simulink model "gm_HDL_pfc_gold_fi_og_vnl"  (R2024b)
settings: Solver=FixedStepDiscrete  StartTime=0.0  StopTime=.2  RelTol=1e-3
InitFcn:
  | fidelity_pfc_vals;
  | nbits=(2^12)-2;
  | load('C:\Users\Angel\Desktop\hil\pfc3ph\matlab\sim\sschdl\pfc_desktop\stateSpaceParameters.mat');
undefined symbols (not defined in the file or in its folder): a, b, c, DiscIntNeverNeededParam, fsw, Gs, s, stateSpaceParameters_1, t_ss, tsw
libraries: simulink x47, hdlmdlgenlib x24, hdlsllib x10, mcbcontrolslib x5, dspsrcs4 x3, slpidlib x2, hdlssclib x2, spsSVPWMGenerator2LevelLib x1, spsPLL3phLib x1, fillib x1
(part 2 of 5)

== system gm_HDL_pfc_gold_fi_og_vnl/Subsystem1/ctrl_pwm/PI_CTRL ==
  id : Inport
  iq : Inport  Port=2
  Add3 : Sum  Inputs=+-
  Add4 : Sum  Inputs=+-
  Constant : Constant  Value=0  SampleTime=t_ss
  Constant1 : Constant  Value=-4  SampleTime=t_ss
  Vd_ctrl : slpidlib/PID Controller  Controller=PI  Form=Parallel  TimeDomain=Discrete-time  UseExternalTs=off  SampleTime=-1  IntegratorMethod=Backward Euler  FilterMethod=Forward Euler  ControllerParametersSource=internal  P=-1.8  I=-.15  UseKiTs=off  D=0  UseExternalDerivativeSource=off  N=100  UseFilter=on  TunerSelectOption=Transfer Function Based (PID Tuner App)  InitialConditionSource=internal  InitialConditionForIntegrator=0  InitialConditionForFilter=0  DifferentiatorICPrevScaledInput=0  ExternalReset=none  TrackingMode=off  Kt=1  LimitOutput=off  SatLimitsSource=internal  UpperSaturationLimit=5e2  LowerSaturationLimit=-5e2  LinearizeAsGain=on  AntiWindupMode=clamping  Kb=1  LimitIntegrator=off  UpperIntegratorSaturationLimit=inf  LowerIntegratorSaturationLimit=-inf  POutMin=[]  POutMax=[]  IOutMin=[]  IOutMax=[]  DOutMin=[]  DOutMax=[]  NOutMin=[]  NOutMax=[]  SumOutMin=[]  SumOutMax=[]  SaturationOutMin=[]  SaturationOutMax=[]  PParamMin=[]  PParamMax=[]  IParamMin=[]  IParamMax=[]  DParamMin=[]  DParamMax=[]  NParamMin=[]  NParamMax=[]  KbParamMin=[]  KbParamMax=[]  KtParamMin=[]  KtParamMax=[]  KbOutMin=[]  KbOutMax=[]  KtOutMin=[]  KtOutMax=[]  IntegratorOutMin=[]  IntegratorOutMax=[]  FilterOutMin=[]  FilterOutMax=[]  SumI1OutMin=[]  SumI1OutMax=[]  SumI2OutMin=[]  SumI2OutMax=[]  SumI3OutMin=[]  SumI3OutMax=[]  SumI4OutMin=[]  SumI4OutMax=[]  SumDOutMin=[]  SumDOutMax=[]  DifferentiatorOutMin=[]  DifferentiatorOutMax=[]  FilterDiffOutCoefMin=[]  FilterDiffOutCoefMax=[]  ReciprocalOutMin=[]  ReciprocalOutMax=[]  SumDenOutMin=[]  SumDenOutMax=[]  SumNumOutMin=[]  SumNumOutMax=[]  DivideOutMin=[]  DivideOutMax=[]  UdiffTsProdOutMin=[]  UdiffTsProdOutMax=[]  NTsProdOutMin=[]  NTsProdOutMax=[]  UintegralTsProdOutMin=[]  UintegralTsProdOutMax=[]  UngainTsProdOutMin=[]  UngainTsProdOutMax=[]  ClampingZeroOutDataTypeStr=Inherit: Inherit via back propagation  ClampingZeroOutMin=[]  ClampingZeroOutMax=[]  FilterDenConstantOutDataTypeStr=Inherit: Inherit via back propagation  FilterDenConstantOutMin=[]  FilterDenConstantOutMax=[]  PCopyOutDataTypeStr=Inherit: Inherit via back propagation  PCopyOutMin=[]  PCopyOutMax=[]  NCopyOutDataTypeStr=Inherit: Inherit via back propagation  NCopyOutMin=[]  NCopyOutMax=[]  IntegratorContinuousStateAttributes=''  IntegratorStateMustResolveToSignalObject=off  IntegratorRTWStateStorageClass=Auto  FilterContinuousStateAttributes=''  FilterStateMustResolveToSignalObject=off  FilterRTWStateStorageClass=Auto  ParallelPVariant=InternalParameters  IdealPVariant=Disabled  IVariant=InternalParameters  DVariant=Disabled  IntegratorVariant=Discrete  SatVariant=Disabled  AWVariant=Passthrough  PCopyVariant=Disabled  TRVariant=Disabled  FdbkBlocksVariant=Forward  IdealPFdbkVariant=Disabled  SatFdbkVariant=Disabled  DerivativeFilterVariant=Disabled  NVariant=Disabled  NCopyVariant=Disabled_SignalSpec  FilterICVariant=Disabled  IntegratorICVariant=InternalICs  ExternalResetVariant=Disabled  TRSumVariant=Passthrough  SumFdbkVariant=Disabled  SumVariant=Sum_PI  TsampFilterVariant=InternalTs  TsampNgainVariant=Passthrough  TsampIntegralVariant=Disabled_SignalSpec  ExternalSaturationOutDataTypeStr=Inherit: Same as second input  DerivativeSourceVariant=Disabled  PreIntVariant=InternalPreInt
  Vq_ctrl : slpidlib/PID Controller  Controller=PI  Form=Parallel  TimeDomain=Discrete-time  UseExternalTs=off  SampleTime=-1  IntegratorMethod=Backward Euler  FilterMethod=Forward Euler  ControllerParametersSource=internal  P=-2  I=-.2  UseKiTs=off  D=0  UseExternalDerivativeSource=off  N=100  UseFilter=on  TunerSelectOption=Transfer Function Based (PID Tuner App)  InitialConditionSource=internal  InitialConditionForIntegrator=0  InitialConditionForFilter=0  DifferentiatorICPrevScaledInput=0  ExternalReset=none  TrackingMode=off  Kt=1  LimitOutput=off  SatLimitsSource=internal  UpperSaturationLimit=5e2  LowerSaturationLimit=-5e2  LinearizeAsGain=on  AntiWindupMode=clamping  Kb=1  LimitIntegrator=off  UpperIntegratorSaturationLimit=inf  LowerIntegratorSaturationLimit=-inf  POutMin=[]  POutMax=[]  IOutMin=[]  IOutMax=[]  DOutMin=[]  DOutMax=[]  NOutMin=[]  NOutMax=[]  SumOutMin=[]  SumOutMax=[]  SaturationOutMin=[]  SaturationOutMax=[]  PParamMin=[]  PParamMax=[]  IParamMin=[]  IParamMax=[]  DParamMin=[]  DParamMax=[]  NParamMin=[]  NParamMax=[]  KbParamMin=[]  KbParamMax=[]  KtParamMin=[]  KtParamMax=[]  KbOutMin=[]  KbOutMax=[]  KtOutMin=[]  KtOutMax=[]  IntegratorOutMin=[]  IntegratorOutMax=[]  FilterOutMin=[]  FilterOutMax=[]  SumI1OutMin=[]  SumI1OutMax=[]  SumI2OutMin=[]  SumI2OutMax=[]  SumI3OutMin=[]  SumI3OutMax=[]  SumI4OutMin=[]  SumI4OutMax=[]  SumDOutMin=[]  SumDOutMax=[]  DifferentiatorOutMin=[]  DifferentiatorOutMax=[]  FilterDiffOutCoefMin=[]  FilterDiffOutCoefMax=[]  ReciprocalOutMin=[]  ReciprocalOutMax=[]  SumDenOutMin=[]  SumDenOutMax=[]  SumNumOutMin=[]  SumNumOutMax=[]  DivideOutMin=[]  DivideOutMax=[]  UdiffTsProdOutMin=[]  UdiffTsProdOutMax=[]  NTsProdOutMin=[]  NTsProdOutMax=[]  UintegralTsProdOutMin=[]  UintegralTsProdOutMax=[]  UngainTsProdOutMin=[]  UngainTsProdOutMax=[]  ClampingZeroOutDataTypeStr=Inherit: Inherit via back propagation  ClampingZeroOutMin=[]  ClampingZeroOutMax=[]  FilterDenConstantOutDataTypeStr=Inherit: Inherit via back propagation  FilterDenConstantOutMin=[]  FilterDenConstantOutMax=[]  PCopyOutDataTypeStr=Inherit: Inherit via back propagation  PCopyOutMin=[]  PCopyOutMax=[]  NCopyOutDataTypeStr=Inherit: Inherit via back propagation  NCopyOutMin=[]  NCopyOutMax=[]  IntegratorContinuousStateAttributes=''  IntegratorStateMustResolveToSignalObject=off  IntegratorRTWStateStorageClass=Auto  FilterContinuousStateAttributes=''  FilterStateMustResolveToSignalObject=off  FilterRTWStateStorageClass=Auto  ParallelPVariant=InternalParameters  IdealPVariant=Disabled  IVariant=InternalParameters  DVariant=Disabled  IntegratorVariant=Discrete  SatVariant=Disabled  AWVariant=Passthrough  PCopyVariant=Disabled  TRVariant=Disabled  FdbkBlocksVariant=Forward  IdealPFdbkVariant=Disabled  SatFdbkVariant=Disabled  DerivativeFilterVariant=Disabled  NVariant=Disabled  NCopyVariant=Disabled_SignalSpec  FilterICVariant=Disabled  IntegratorICVariant=InternalICs  ExternalResetVariant=Disabled  TRSumVariant=Passthrough  SumFdbkVariant=Disabled  SumVariant=Sum_PI  TsampFilterVariant=InternalTs  TsampNgainVariant=Passthrough  TsampIntegralVariant=Disabled_SignalSpec  ExternalSaturationOutDataTypeStr=Inherit: Same as second input  DerivativeSourceVariant=Disabled  PreIntVariant=InternalPreInt
  Vd_inductor : Outport
  Vq_inductor : Outport  Port=2
  wires:
  Add3/1 -> Vd_ctrl/1  "error_id"
  id/1 -> Add3/2
  Constant/1 -> Add3/1
  iq/1 -> Add4/2
  Add4/1 -> Vq_ctrl/1  "error_iq"
  Vd_ctrl/1 -> Vd_inductor/1
  Vq_ctrl/1 -> Vq_inductor/1
  Constant1/1 -> Add4/1

== system gm_HDL_pfc_gold_fi_og_vnl/Subsystem1/ctrl_pwm/SVPWM ==
  Vd_inductor : Inport
  angle : Inport  Port=2
  Vq_inductor : Inport  Port=3
  Cos : Trigonometry  Operator=cos
  Inverse Park Transform : mcbcontrolslib/Inverse Park Transform  PhaseInput=Two inputs  AxisAlignment=D-axis  ThetaInput=Sine and Cosine electrical position  AngleInput=Per-unit  N_points=1024
  SVPWM Generator (2-Level) : spsSVPWMGenerator2LevelLib/SVPWM Generator (2-Level)  InputType=alpha-beta components  SwitchingPattern=Pattern #1  Fc=fsw*1e3  ParUref=[0.8 -30 50]  Ts=t_ss
  Sin : Trigonometry
  P : Outport
  wires:
  Vd_inductor/1 -> Inverse Park Transform/1
  Vq_inductor/1 -> Inverse Park Transform/2
  Inverse Park Transform/2 -> SVPWM Generator (2-Level)/2  "Vbet_indc"
  Sin/1 -> Inverse Park Transform/3
  Cos/1 -> Inverse Park Transform/4
  Inverse Park Transform/1 -> SVPWM Generator (2-Level)/1  "Valp_indc"
  angle/1 -> Cos/1, Sin/1
  SVPWM Generator (2-Level)/1 -> P/1

== system gm_HDL_pfc_gold_fi_og_vnl/Subsystem1/ctrl_pwm/transforms ==
  a : Inport
  b : Inport  Port=2
  In3 : Inport  Port=3
  In4 : Inport  Port=4
  In5 : Inport  Port=5
  Claro-Parl Transform : Subsystem  Commented=on
  Claro-Parl Transform1 : Subsystem
  Delay : Delay  DelayLength=1
  Delay1 : Delay  DelayLength=1
  Mux : Mux  Inputs=3
  PLL (3ph) : spsPLL3phLib/PLL (3ph)  Fmin=50  Par_Init=[0, 50]  ParK=[180,3200,1]  TcD=1e-4  MaxRateChangeFreq=12  FilterCutOffFreq=25  Ts=t_ss  AGC=on
  Terminator : Terminator
  id : Outport
  iq : Outport  Port=2
  angle : Outport  Port=3
  wires:
  Mux/1 -> PLL (3ph)/1
  PLL (3ph)/2 -> angle/1, Claro-Parl Transform1/3(wt), Claro-Parl Transform/3(wt)  "angle"
  PLL (3ph)/1 -> Terminator/1
  In3/1 -> Mux/1, Claro-Parl Transform/1(a)
  In5/1 -> Mux/3
  b/1 -> Delay1/1
  In4/1 -> Claro-Parl Transform/2(b), Mux/2
  a/1 -> Delay/1
  Delay/1 -> Claro-Parl Transform1/1(a)
  Delay1/1 -> Claro-Parl Transform1/2(b)
  Claro-Parl Transform/1(d) -> ?  "vd"
  Claro-Parl Transform/2(q) -> ?  "vq"
  Claro-Parl Transform1/1(d) -> id/1  "id"
  Claro-Parl Transform1/2(q) -> iq/1  "iq"

== system gm_HDL_pfc_gold_fi_og_vnl/simscape_system/simscape_system/FET_CTRL ==
  vs : Inport  OutDataTypeStr=fixdt(1, 18, 6)  PortDimensions=[6]  SampleTime=1.38600138600139e-08
  is : Inport  Port=2  OutDataTypeStr=fixdt(1, 18, 6)  PortDimensions=[6]  SampleTime=1.38600138600139e-08
  G : Inport  Port=3  OutDataTypeStr=boolean  PortDimensions=[6]  SampleTime=1.38600138600139e-08
  sch_ctr_36 : Inport  Port=4  OutDataTypeStr=fixdt(0, 6, 0)  SampleTime=1.38600138600139e-08
  Discrete-Time Integrator_reg : RateTransition  InitialCondition=double(0)  OutPortSampleTimeOpt=Multiple of input port sample time  OutPortSampleTimeMultiple=37
  Discrete-Time Integrator_reg_absorbed : Delay  DelayLength=0
  crp_temp_streamed : Subsystem
  in0_repeat : RateTransition  Integrity=off  Deterministic=off  OutPortSampleTimeOpt=Multiple of input port sample time  OutPortSampleTimeMultiple=1/37
  ic : Outport  SampleTime=1.38600138600139e-08
  wires:
  Discrete-Time Integrator_reg_absorbed/1 -> in0_repeat/1
  crp_temp_streamed/2(out1) -> ic/1
  sch_ctr_36/1 -> crp_temp_streamed/5(enb_counter)
  Discrete-Time Integrator_reg/1 -> Discrete-Time Integrator_reg_absorbed/1
  is/1 -> crp_temp_streamed/4(in3)
  vs/1 -> crp_temp_streamed/3(in2)
  crp_temp_streamed/1(out0) -> Discrete-Time Integrator_reg/1
  in0_repeat/1 -> crp_temp_streamed/1(in0)
  G/1 -> crp_temp_streamed/2(in1)

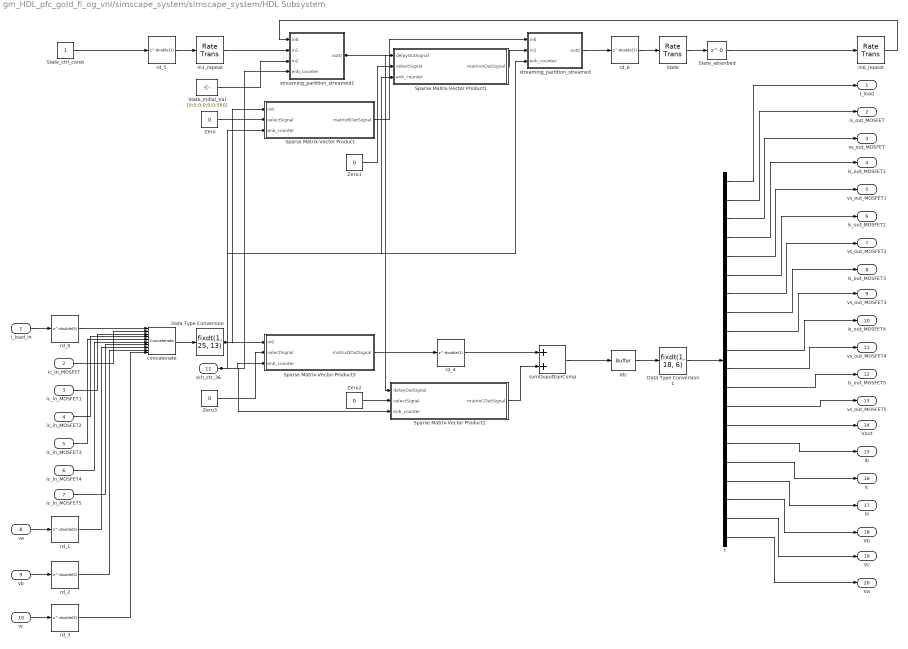
== system gm_HDL_pfc_gold_fi_og_vnl/simscape_system/simscape_system/HDL Subsystem ==
  I_load_in : Inport  OutDataTypeStr=fixdt(1, 18, 8)  PortDimensions=1  SampleTime=1.38600138600139e-08
  ic_in_MOSFET : Inport  Port=2  OutDataTypeStr=fixdt(1, 18, 8)  PortDimensions=1  SampleTime=1.38600138600139e-08
  ic_in_MOSFET1 : Inport  Port=3  OutDataTypeStr=fixdt(1, 18, 8)  PortDimensions=1  SampleTime=1.38600138600139e-08
  ic_in_MOSFET2 : Inport  Port=4  OutDataTypeStr=fixdt(1, 18, 8)  PortDimensions=1  SampleTime=1.38600138600139e-08
  ic_in_MOSFET3 : Inport  Port=5  OutDataTypeStr=fixdt(1, 18, 8)  PortDimensions=1  SampleTime=1.38600138600139e-08
  ic_in_MOSFET4 : Inport  Port=6  OutDataTypeStr=fixdt(1, 18, 8)  PortDimensions=1  SampleTime=1.38600138600139e-08
  ic_in_MOSFET5 : Inport  Port=7  OutDataTypeStr=fixdt(1, 18, 8)  PortDimensions=1  SampleTime=1.38600138600139e-08
  va : Inport  Port=8  OutDataTypeStr=fixdt(1, 18, 8)  PortDimensions=1  SampleTime=1.38600138600139e-08
  vb : Inport  Port=9  OutDataTypeStr=fixdt(1, 18, 8)  PortDimensions=1  SampleTime=1.38600138600139e-08
  vc : Inport  Port=10  OutDataTypeStr=fixdt(1, 18, 8)  PortDimensions=1  SampleTime=1.38600138600139e-08
  sch_ctr_36 : Inport  Port=11  OutDataTypeStr=fixdt(0, 6, 0)  SampleTime=1.38600138600139e-08
  Data Type Conversion : DataTypeConversion  OutDataTypeStr=fixdt(1, 25, 13)  SampleTime=1.38600138600139e-08  SaturateOnIntegerOverflow=off  RndMeth=Floor
  Data Type Conversion1 : DataTypeConversion  OutDataTypeStr=fixdt(1, 18, 6)  SampleTime=1.38600138600139e-08  SaturateOnIntegerOverflow=off  RndMeth=Floor
  Sparse Matrix-Vector Product : Subsystem
  Sparse Matrix-Vector Product1 : Subsystem
  Sparse Matrix-Vector Product2 : Subsystem
  Sparse Matrix-Vector Product3 : Subsystem
  State : RateTransition  InitialCondition=double(0)  OutPortSampleTimeOpt=Multiple of input port sample time  OutPortSampleTimeMultiple=37
  State_Initial_Val : Constant  Value=[0;0;0;0;0;0;580]  OutDataTypeStr=fixdt(1, 25, 13)  SampleTime=1.38600138600139e-08
  State_absorbed : Delay  DelayLength=0
  State_ctrl_const : Constant  OutDataTypeStr=boolean  SampleTime=5.12820512820513e-07
  Zero{,1..3} (4 alike) : Constant  Value=0  OutDataTypeStr=boolean  SampleTime=1.38600138600139e-08
  concatenate : Concatenate  NumInputs=10
  dtc : hdlmdlgenlib/Buffer
  in0_repeat : RateTransition  Integrity=off  Deterministic=off  OutPortSampleTimeOpt=Multiple of input port sample time  OutPortSampleTimeMultiple=1/37
  in1_repeat : RateTransition  Integrity=off  Deterministic=off  OutPortSampleTimeOpt=Multiple of input port sample time  OutPortSampleTimeMultiple=1/37
  rd_{0..3} (4 alike) : Delay  DelayLength=double(5)  InitialCondition=0  SampleTime=1.38600138600139e-08
  rd_4 : Delay  DelayLength=double(1)  InitialCondition=0  SampleTime=1.38600138600139e-08
  rd_5 : Delay  DelayLength=double(1)  InitialCondition=0  SampleTime=5.12820512820513e-07
  rd_6 : Delay  DelayLength=double(1)  InitialCondition=0  SampleTime=1.38600138600139e-08
  streaming_partition_streamed : Subsystem
  streaming_partition_streamed1 : Subsystem
  sumOuputEqnComp : Sum  OutDataTypeStr=fixdt(1, 25, 13)  SampleTime=1.38600138600139e-08
  t : Demux  Outputs=20
  I_load : Outport  SampleTime=1.38600138600139e-08
  is_out_MOSFET : Outport  Port=2  SampleTime=1.38600138600139e-08
  vs_out_MOSFET : Outport  Port=3  SampleTime=1.38600138600139e-08
  is_out_MOSFET1 : Outport  Port=4  SampleTime=1.38600138600139e-08
  vs_out_MOSFET1 : Outport  Port=5  SampleTime=1.38600138600139e-08
  is_out_MOSFET2 : Outport  Port=6  SampleTime=1.38600138600139e-08
  vs_out_MOSFET2 : Outport  Port=7  SampleTime=1.38600138600139e-08
  is_out_MOSFET3 : Outport  Port=8  SampleTime=1.38600138600139e-08
  vs_out_MOSFET3 : Outport  Port=9  SampleTime=1.38600138600139e-08
  is_out_MOSFET4 : Outport  Port=10  SampleTime=1.38600138600139e-08
  vs_out_MOSFET4 : Outport  Port=11  SampleTime=1.38600138600139e-08
  is_out_MOSFET5 : Outport  Port=12  SampleTime=1.38600138600139e-08
  vs_out_MOSFET5 : Outport  Port=13  SampleTime=1.38600138600139e-08
  Vout : Outport  Port=14  SampleTime=1.38600138600139e-08
  Ib : Outport  Port=15  SampleTime=1.38600138600139e-08
  Ic : Outport  Port=16  SampleTime=1.38600138600139e-08
  Ia : Outport  Port=17  SampleTime=1.38600138600139e-08
  Vb : Outport  Port=18  SampleTime=1.38600138600139e-08
  Vc : Outport  Port=19  SampleTime=1.38600138600139e-08
  Va : Outport  Port=20  SampleTime=1.38600138600139e-08
  wires:
  in0_repeat/1 -> streaming_partition_streamed1/1(in0)
  t/14 -> Vout/1
  t/6 -> is_out_MOSFET2/1
  t/3 -> vs_out_MOSFET/1
  t/1 -> I_load/1
  State_absorbed/1 -> in0_repeat/1
  Data Type Conversion1/1 -> t/1
  State/1 -> State_absorbed/1
  dtc/1 -> Data Type Conversion1/1
  sumOuputEqnComp/1 -> dtc/1
  t/15 -> Ib/1
  rd_4/1 -> sumOuputEqnComp/1
  Sparse Matrix-Vector Product2/1(matrixCOutSignal) -> sumOuputEqnComp/2
  Sparse Matrix-Vector Product1/1(matrixAOutSignal) -> streaming_partition_streamed/2(in1)
  Zero2/1 -> Sparse Matrix-Vector Product2/2(selectSignal)
  Sparse Matrix-Vector Product/1(matrixBOutSignal) -> streaming_partition_streamed/1(in0)
  streaming_partition_streamed1/1(out0) -> Sparse Matrix-Vector Product2/1(delayOutSignal), Sparse Matrix-Vector Product1/1(delayOutSignal)
  Zero3/1 -> Sparse Matrix-Vector Product3/2(selectSignal)
  Data Type Conversion/1 -> Sparse Matrix-Vector Product/1(in0), Sparse Matrix-Vector Product3/1(in0)
  t/12 -> is_out_MOSFET5/1
  t/16 -> Ic/1
  Zero/1 -> Sparse Matrix-Vector Product/2(selectSignal)
  in1_repeat/1 -> streaming_partition_streamed1/2(in1)
  t/8 -> is_out_MOSFET3/1
  concatenate/1 -> Data Type Conversion/1
  t/2 -> is_out_MOSFET/1
  t/20 -> Va/1
  rd_5/1 -> in1_repeat/1
  rd_3/1 -> concatenate/10
  rd_2/1 -> concatenate/9
  t/18 -> Vb/1
  rd_1/1 -> concatenate/8
  t/19 -> Vc/1
  ic_in_MOSFET5/1 -> concatenate/7
  Zero1/1 -> Sparse Matrix-Vector Product1/2(selectSignal)
  ic_in_MOSFET4/1 -> concatenate/6
  streaming_partition_streamed/1(out0) -> rd_6/1
  ic_in_MOSFET3/1 -> concatenate/5
  ic_in_MOSFET2/1 -> concatenate/4
  Sparse Matrix-Vector Product3/1(matrixDOutSignal) -> rd_4/1
  ic_in_MOSFET1/1 -> concatenate/3
  sch_ctr_36/1 -> streaming_partition_streamed/3(enb_counter), Sparse Matrix-Vector Product/3(enb_counter), Sparse Matrix-Vector Product2/3(enb_counter), streaming_partition_streamed1/4(enb_counter), Sparse Matrix-Vector Product3/3(enb_counter), Sparse Matrix-Vector Product1/3(enb_counter)
  rd_6/1 -> State/1
  t/13 -> vs_out_MOSFET5/1
  t/17 -> Ia/1
  rd_0/1 -> concatenate/1
  ic_in_MOSFET/1 -> concatenate/2
  t/4 -> is_out_MOSFET1/1
  t/10 -> is_out_MOSFET4/1
  vc/1 -> rd_3/1
  State_Initial_Val/1 -> streaming_partition_streamed1/3(in2)
  va/1 -> rd_1/1
  t/9 -> vs_out_MOSFET3/1
  I_load_in/1 -> rd_0/1
  t/5 -> vs_out_MOSFET1/1
  t/7 -> vs_out_MOSFET2/1
  t/11 -> vs_out_MOSFET4/1
  vb/1 -> rd_2/1
  State_ctrl_const/1 -> rd_5/1

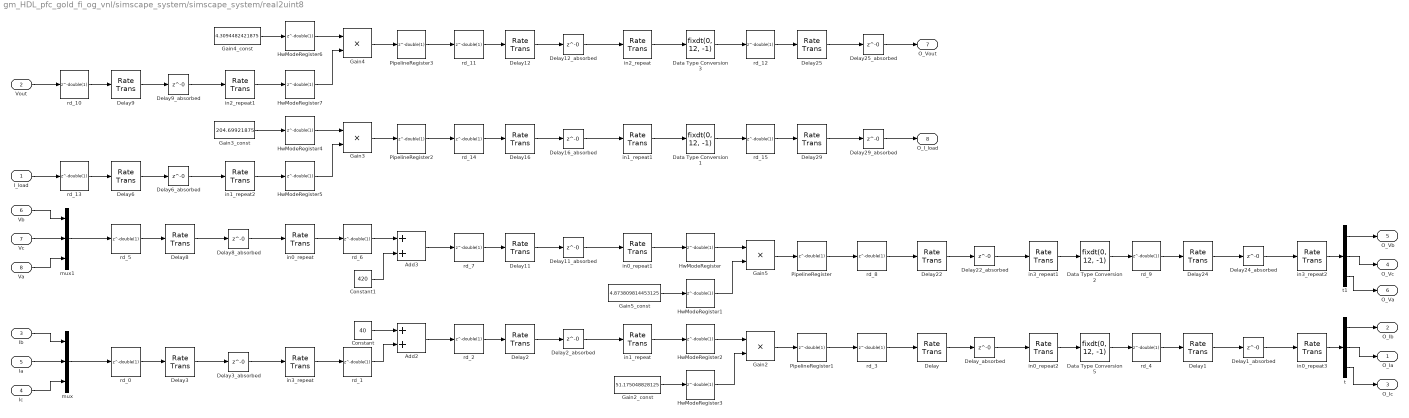
== system gm_HDL_pfc_gold_fi_og_vnl/simscape_system/simscape_system/real2uint8 ==
  I_load : Inport  OutDataTypeStr=fixdt(1, 18, 6)  PortDimensions=1  SampleTime=1.38600138600139e-08
  Vout : Inport  Port=2  OutDataTypeStr=fixdt(1, 18, 6)  PortDimensions=1  SampleTime=1.38600138600139e-08
  Ib : Inport  Port=3  OutDataTypeStr=fixdt(1, 18, 6)  PortDimensions=1  SampleTime=1.38600138600139e-08
  Ic : Inport  Port=4  OutDataTypeStr=fixdt(1, 18, 6)  PortDimensions=1  SampleTime=1.38600138600139e-08
  Ia : Inport  Port=5  OutDataTypeStr=fixdt(1, 18, 6)  PortDimensions=1  SampleTime=1.38600138600139e-08
  Vb : Inport  Port=6  OutDataTypeStr=fixdt(1, 18, 6)  PortDimensions=1  SampleTime=1.38600138600139e-08
  Vc : Inport  Port=7  OutDataTypeStr=fixdt(1, 18, 6)  PortDimensions=1  SampleTime=1.38600138600139e-08
  Va : Inport  Port=8  OutDataTypeStr=fixdt(1, 18, 6)  PortDimensions=1  SampleTime=1.38600138600139e-08
  Add2 : Sum  OutDataTypeStr=fixdt(1, 19, 6)  AccumDataTypeStr=fixdt(1, 19, 6)  SampleTime=1.38600138600139e-08
  Add3 : Sum  OutDataTypeStr=fixdt(1, 19, 6)  AccumDataTypeStr=fixdt(1, 19, 6)  SampleTime=1.38600138600139e-08
  Constant : Constant  Value=40  OutDataTypeStr=fixdt(1, 18, 6)  SampleTime=1.38600138600139e-08
  Constant1 : Constant  Value=420  OutDataTypeStr=fixdt(1, 18, 6)  SampleTime=1.38600138600139e-08
  Data Type Conversion{1..3,5} (4 alike) : DataTypeConversion  OutDataTypeStr=fixdt(0, 12, -1)  SampleTime=1.38600138600139e-08  SaturateOnIntegerOverflow=off  RndMeth=Floor
  Delay{,1..3,6,8..9,11..12,16,22,24..25,29} (14 alike) : RateTransition  InitialCondition=double(0)  OutPortSampleTimeOpt=Multiple of input port sample time  OutPortSampleTimeMultiple=37
  Delay11_absorbed : Delay  DelayLength=0
  Delay12_absorbed : Delay  DelayLength=0
  Delay16_absorbed : Delay  DelayLength=0
  Delay1_absorbed : Delay  DelayLength=0
  Delay22_absorbed : Delay  DelayLength=0
  Delay24_absorbed : Delay  DelayLength=0
  Delay25_absorbed : Delay  DelayLength=0
  Delay29_absorbed : Delay  DelayLength=0
  Delay2_absorbed : Delay  DelayLength=0
  Delay3_absorbed : Delay  DelayLength=0
  Delay6_absorbed : Delay  DelayLength=0
  Delay8_absorbed : Delay  DelayLength=0
  Delay9_absorbed : Delay  DelayLength=0
  Delay_absorbed : Delay  DelayLength=0
  Gain2 : Product  Inputs=**  OutDataTypeStr=fixdt(1, 38, 18)  SampleTime=1.38600138600139e-08
  Gain2_const : Constant  Value=51.175048828125  OutDataTypeStr=fixdt(1, 19, 12)  SampleTime=1.38600138600139e-08
  Gain3 : Product  Inputs=**  OutDataTypeStr=fixdt(1, 36, 15)  SampleTime=1.38600138600139e-08
  Gain3_const : Constant  Value=204.69921875  OutDataTypeStr=fixdt(1, 18, 9)  SampleTime=1.38600138600139e-08
  Gain4 : Product  Inputs=**  OutDataTypeStr=fixdt(1, 36, 20)  SampleTime=1.38600138600139e-08
  Gain4_const : Constant  Value=4.3094482421875  OutDataTypeStr=fixdt(1, 18, 14)  SampleTime=1.38600138600139e-08
  Gain5 : Product  Inputs=**  OutDataTypeStr=fixdt(1, 38, 21)  SampleTime=1.38600138600139e-08
  Gain5_const : Constant  Value=4.873809814453125  OutDataTypeStr=fixdt(1, 19, 15)  SampleTime=1.38600138600139e-08
  HwModeRegister{,1..7} (8 alike) : Delay  DelayLength=double(1)  InitialCondition=0  SampleTime=1.38600138600139e-08
  PipelineRegister{,1..3} (4 alike) : Delay  DelayLength=double(1)  InitialCondition=0  SampleTime=1.38600138600139e-08
  in0_repeat{,1..3} (4 alike) : RateTransition  Integrity=off  Deterministic=off  OutPortSampleTimeOpt=Multiple of input port sample time  OutPortSampleTimeMultiple=1/37
  in1_repeat : RateTransition  Integrity=off  Deterministic=off  OutPortSampleTimeOpt=Multiple of input port sample time  OutPortSampleTimeMultiple=1/37
  in1_repeat1 : RateTransition  Integrity=off  Deterministic=off  OutPortSampleTimeOpt=Multiple of input port sample time  OutPortSampleTimeMultiple=1/37
  in1_repeat2 : RateTransition  Integrity=off  Deterministic=off  OutPortSampleTimeOpt=Multiple of input port sample time  OutPortSampleTimeMultiple=1/37
  in2_repeat : RateTransition  Integrity=off  Deterministic=off  OutPortSampleTimeOpt=Multiple of input port sample time  OutPortSampleTimeMultiple=1/37
  in2_repeat1 : RateTransition  Integrity=off  Deterministic=off  OutPortSampleTimeOpt=Multiple of input port sample time  OutPortSampleTimeMultiple=1/37
  in3_repeat : RateTransition  Integrity=off  Deterministic=off  OutPortSampleTimeOpt=Multiple of input port sample time  OutPortSampleTimeMultiple=1/37
  in3_repeat1 : RateTransition  Integrity=off  Deterministic=off  OutPortSampleTimeOpt=Multiple of input port sample time  OutPortSampleTimeMultiple=1/37
  in3_repeat2 : RateTransition  Integrity=off  Deterministic=off  OutPortSampleTimeOpt=Multiple of input port sample time  OutPortSampleTimeMultiple=1/37
  mux : Mux  Inputs=3
  mux1 : Mux  Inputs=3
  rd_{0..15} (16 alike) : Delay  DelayLength=double(1)  InitialCondition=0  SampleTime=1.38600138600139e-08
  t : Demux  Outputs=3
  t1 : Demux  Outputs=3
  O_Ia : Outport  SampleTime=1.38600138600139e-08
  O_Ib : Outport  Port=2  SampleTime=1.38600138600139e-08
  O_Ic : Outport  Port=3  SampleTime=1.38600138600139e-08
  O_Vc : Outport  Port=4  SampleTime=1.38600138600139e-08
  O_Vb : Outport  Port=5  SampleTime=1.38600138600139e-08
  O_Va : Outport  Port=6  SampleTime=1.38600138600139e-08
  O_Vout : Outport  Port=7  SampleTime=5.12820512820513e-07
  O_I_load : Outport  Port=8  SampleTime=5.12820512820513e-07
  wires:
  t/3 -> O_Ic/1
  t/2 -> O_Ia/1
  t/1 -> O_Ib/1
  t1/3 -> O_Va/1
  t1/2 -> O_Vc/1
  t1/1 -> O_Vb/1
  in0_repeat3/1 -> t/1
  Delay1_absorbed/1 -> in0_repeat3/1
  Delay24_absorbed/1 -> in3_repeat2/1
  rd_4/1 -> Delay1/1
  rd_9/1 -> Delay24/1
  Data Type Conversion5/1 -> rd_4/1
  Data Type Conversion2/1 -> rd_9/1
  in0_repeat2/1 -> Data Type Conversion5/1
  in3_repeat1/1 -> Data Type Conversion2/1
  Delay_absorbed/1 -> in0_repeat2/1
  Delay22_absorbed/1 -> in3_repeat1/1
  Delay/1 -> Delay_absorbed/1
  Delay22/1 -> Delay22_absorbed/1
  rd_3/1 -> Delay/1
  rd_8/1 -> Delay22/1
  Delay29_absorbed/1 -> O_I_load/1
  Delay25_absorbed/1 -> O_Vout/1
  PipelineRegister1/1 -> rd_3/1
  Delay29/1 -> Delay29_absorbed/1
  Delay25/1 -> Delay25_absorbed/1
  Gain2/1 -> PipelineRegister1/1
  Gain5/1 -> PipelineRegister/1
  rd_15/1 -> Delay29/1
  rd_12/1 -> Delay25/1
  HwModeRegister2/1 -> Gain2/1
  HwModeRegister/1 -> Gain5/1
  Data Type Conversion3/1 -> rd_12/1
  Gain2_const/1 -> HwModeRegister3/1
  in2_repeat/1 -> Data Type Conversion3/1
  Gain5_const/1 -> HwModeRegister1/1
  Delay11_absorbed/1 -> in0_repeat1/1
  Data Type Conversion1/1 -> rd_15/1
  Delay12_absorbed/1 -> in2_repeat/1
  Delay2/1 -> Delay2_absorbed/1
  Delay16/1 -> Delay16_absorbed/1
  Delay1/1 -> Delay1_absorbed/1
  rd_11/1 -> Delay12/1
  in1_repeat/1 -> HwModeRegister2/1
  Add3/1 -> rd_7/1
  rd_1/1 -> Add2/2
  Delay2_absorbed/1 -> in1_repeat/1
  Constant/1 -> Add2/1
  Delay24/1 -> Delay24_absorbed/1
  rd_6/1 -> Add3/1
  Gain4/1 -> PipelineRegister3/1
  rd_14/1 -> Delay16/1
  in3_repeat/1 -> rd_1/1
  in0_repeat/1 -> rd_6/1
  HwModeRegister1/1 -> Gain5/2
  HwModeRegister5/1 -> Gain3/2
  HwModeRegister4/1 -> Gain3/1
  HwModeRegister6/1 -> Gain4/1
  PipelineRegister2/1 -> rd_14/1
  in0_repeat1/1 -> HwModeRegister/1
  Delay8_absorbed/1 -> in0_repeat/1
  Gain3_const/1 -> HwModeRegister4/1
  rd_7/1 -> Delay11/1
  Gain4_const/1 -> HwModeRegister6/1
  in1_repeat1/1 -> Data Type Conversion1/1
  Delay3/1 -> Delay3_absorbed/1
  Delay8/1 -> Delay8_absorbed/1
  Delay9_absorbed/1 -> in2_repeat1/1
  Constant1/1 -> Add3/2
  Add2/1 -> rd_2/1
  in1_repeat2/1 -> HwModeRegister5/1
  rd_0/1 -> Delay3/1
  Delay12/1 -> Delay12_absorbed/1
  rd_5/1 -> Delay8/1
  rd_2/1 -> Delay2/1
  Delay9/1 -> Delay9_absorbed/1
  mux/1 -> rd_0/1
  Delay6/1 -> Delay6_absorbed/1
  PipelineRegister3/1 -> rd_11/1
  mux1/1 -> rd_5/1
  Delay3_absorbed/1 -> in3_repeat/1
  rd_13/1 -> Delay6/1
  rd_10/1 -> Delay9/1
  HwModeRegister3/1 -> Gain2/2
  Gain3/1 -> PipelineRegister2/1
  in3_repeat2/1 -> t1/1
  Delay6_absorbed/1 -> in1_repeat2/1
  Delay11/1 -> Delay11_absorbed/1
  Vb/1 -> mux1/1
  Vc/1 -> mux1/2
  PipelineRegister/1 -> rd_8/1
  Va/1 -> mux1/3
  Delay16_absorbed/1 -> in1_repeat1/1
  Ia/1 -> mux/2
  Vout/1 -> rd_10/1
  I_load/1 -> rd_13/1
  HwModeRegister7/1 -> Gain4/2
  Ib/1 -> mux/1
  in2_repeat1/1 -> HwModeRegister7/1
  Ic/1 -> mux/3

== system gm_HDL_pfc_gold_fi_og_vnl/simscape_system_vnl/HDL Subsystem/HDL Algorithm ==
  In1 : Inport
  Delay1 : Delay  DelayLength=1
  Delay2 : Delay
  Output : Subsystem
  Sel : Constant  Value=0  OutDataTypeStr=uint32  SampleTime=-1
  State Delay : Delay  DelayLength=1  InitialCondition=single(stateSpaceParameters_1.X0)
  State Switch : Switch  Criteria=u2 ~= 0  SaturateOnIntegerOverflow=off  InputSameDT=off
  State Update : Subsystem
  Valid Out : Constant  OutDataTypeStr=boolean  SampleTime=4.395604395604395e-07
  X0 : Constant  Value=single(stateSpaceParameters_1.X0)  SampleTime=4.395604395604395e-07
  Out1 : Outport  VectorParamsAs1DForOutWhenUnconnected=off
  wires:
  In1/1 -> State Update/1(In1), Delay1/1
  State Switch/1 -> State Update/2(State), Output/2(State)
  Output/1(Out1) -> Out1/1
  X0/1 -> State Switch/3
  Delay2/1 -> State Switch/2
  State Delay/1 -> State Switch/1
  Valid Out/1 -> Delay2/1
  State Update/1(State Out) -> State Delay/1
  Sel/1 -> State Update/3(Sel), Output/3(Sel)
  Delay1/1 -> Output/1(In1)

== system gm_HDL_pfc_gold_fi_og_vnl/Subsystem1/ctrl_pwm/transforms/Claro-Parl Transform ==
  a : Inport
  b : Inport  Port=2
  wt : Inport  Port=3
  Clarke Transform : mcbcontrolslib/Clarke Transform  VariantControl=Variant2  PhaseInput=Two inputs  EnPowerInv=off
  Cos : Trigonometry  Operator=cos
  Park Transform : mcbcontrolslib/Park Transform  PhaseInput=Two inputs  AxisAlignment=D-axis  ThetaInput=Sine and Cosine electrical position  AngleInput=Per-unit  N_points=1024
  Sin : Trigonometry
  d : Outport
  q : Outport  Port=2
  wires:
  Clarke Transform/2 -> Park Transform/2  "Vbet_sourc"
  b/1 -> Clarke Transform/2
  Park Transform/2 -> q/1
  Park Transform/1 -> d/1
  Clarke Transform/1 -> Park Transform/1  "Valp_sourc"
  wt/1 -> Cos/1, Sin/1
  a/1 -> Clarke Transform/1
  Sin/1 -> Park Transform/3
  Cos/1 -> Park Transform/4

== system gm_HDL_pfc_gold_fi_og_vnl/Subsystem1/ctrl_pwm/transforms/Claro-Parl Transform1 ==
  a : Inport
  b : Inport  Port=2
  wt : Inport  Port=3
  Clarke Transform : mcbcontrolslib/Clarke Transform  VariantControl=Variant2  PhaseInput=Two inputs  EnPowerInv=off
  Cos : Trigonometry  Operator=cos
  Park Transform : mcbcontrolslib/Park Transform  PhaseInput=Two inputs  AxisAlignment=D-axis  ThetaInput=Sine and Cosine electrical position  AngleInput=Per-unit  N_points=1024
  Sin : Trigonometry
  d : Outport
  q : Outport  Port=2
  wires:
  Clarke Transform/2 -> Park Transform/2  "Ibet_sourc"
  b/1 -> Clarke Transform/2
  Park Transform/2 -> q/1
  Park Transform/1 -> d/1
  Clarke Transform/1 -> Park Transform/1  "Ialp_sourc"
  wt/1 -> Cos/1, Sin/1
  a/1 -> Clarke Transform/1
  Sin/1 -> Park Transform/3
  Cos/1 -> Park Transform/4

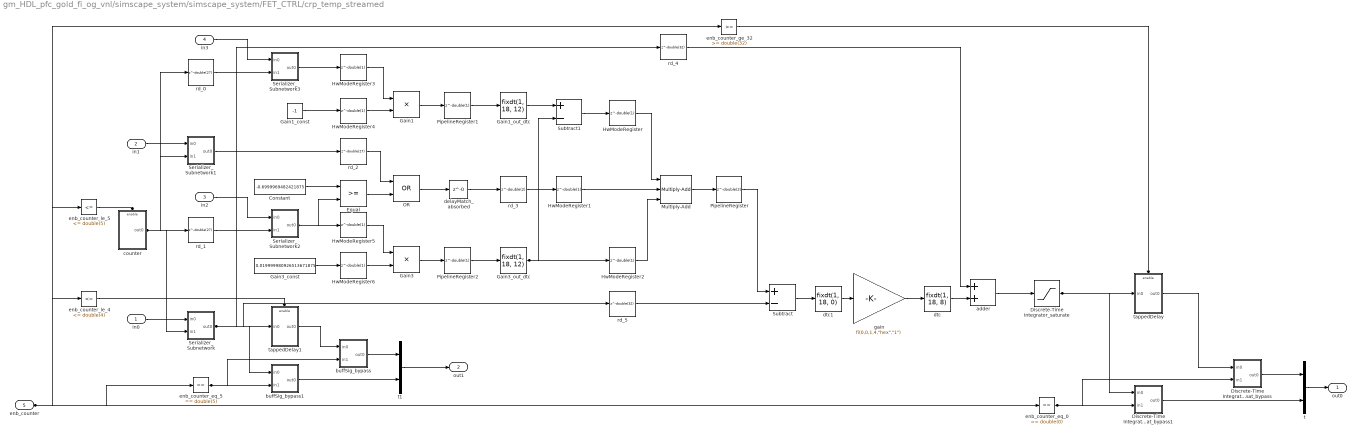
== system gm_HDL_pfc_gold_fi_og_vnl/simscape_system/simscape_system/FET_CTRL/crp_temp_streamed ==
  in0 : Inport  OutDataTypeStr=fixdt(1, 18, 8)  PortDimensions=[6]  SampleTime=1.38600138600139e-08
  in1 : Inport  Port=2  OutDataTypeStr=boolean  PortDimensions=[6]  SampleTime=1.38600138600139e-08
  in2 : Inport  Port=3  OutDataTypeStr=fixdt(1, 18, 6)  PortDimensions=[6]  SampleTime=1.38600138600139e-08
  in3 : Inport  Port=4  OutDataTypeStr=fixdt(1, 18, 6)  PortDimensions=[6]  SampleTime=1.38600138600139e-08
  enb_counter : Inport  Port=5  OutDataTypeStr=fixdt(0, 6, 0)  SampleTime=1.38600138600139e-08
  Constant : Constant  Value=-0.6999969482421875  OutDataTypeStr=fixdt(1, 18, 17)  SampleTime=1.38600138600139e-08
  Discrete-Time Integrator_saturate : Saturate  UpperLimit="fi(0,1,18,8,\"hex\",\"06400\")"  LowerLimit="fi(0,1,18,8,\"hex\",\"39c00\")"  SampleTime=1.38600138600139e-08  OutDataTypeStr=fixdt(1, 18, 8)
  Discrete-Time Integrator_u_sat_bypass : Subsystem
  Discrete-Time Integrator_u_sat_bypass1 : Subsystem
  Equal : RelationalOperator  OutDataTypeStr=boolean  SampleTime=1.38600138600139e-08  InputSameDT=off
  Gain1 : Product  Inputs=**  OutDataTypeStr=fixdt(1, 36, 23)  SampleTime=1.38600138600139e-08
  Gain1_const : Constant  Value=-1  OutDataTypeStr=fixdt(1, 18, 17)  SampleTime=1.38600138600139e-08
  Gain1_out_dtc : DataTypeConversion  OutDataTypeStr=fixdt(1, 18, 12)  SampleTime=1.38600138600139e-08  SaturateOnIntegerOverflow=off  RndMeth=Floor
  Gain3 : Product  Inputs=**  OutDataTypeStr=fixdt(1, 36, 28)  SampleTime=1.38600138600139e-08
  Gain3_const : Constant  Value=0.019999980926513671875  OutDataTypeStr=fixdt(1, 18, 22)  SampleTime=1.38600138600139e-08
  Gain3_out_dtc : DataTypeConversion  OutDataTypeStr=fixdt(1, 18, 12)  SampleTime=1.38600138600139e-08  SaturateOnIntegerOverflow=off  RndMeth=Floor
  HwModeRegister{,1..6} (7 alike) : Delay  DelayLength=double(1)  InitialCondition=0  SampleTime=1.38600138600139e-08
  Multiply-Add : hdlsllib/HDL Operations/Multiply-Add  Function=c+(a.*b)  datatype=fixdt(1, 18, 12)  DoSatur=on  FMA=off
  OR : Logic  Operator=OR  AllPortsSameDT=off  OutDataTypeStr=boolean  SampleTime=1.38600138600139e-08
  PipelineRegister : Delay  DelayLength=double(2)  InitialCondition=0  SampleTime=1.38600138600139e-08
  PipelineRegister1 : Delay  DelayLength=double(1)  InitialCondition=0  SampleTime=1.38600138600139e-08
  PipelineRegister2 : Delay  DelayLength=double(1)  InitialCondition=0  SampleTime=1.38600138600139e-08
  Serializer_Subnetwork : Subsystem
  Serializer_Subnetwork1 : Subsystem
  Serializer_Subnetwork2 : Subsystem
  Serializer_Subnetwork3 : Subsystem
  Subtract : Sum  Inputs=+-  OutDataTypeStr=fixdt(1, 18, 12)  AccumDataTypeStr=fixdt(1, 23, 12)  SampleTime=1.38600138600139e-08
  Subtract1 : Sum  Inputs=+-  OutDataTypeStr=fixdt(1, 18, 11)  AccumDataTypeStr=fixdt(1, 19, 12)  SampleTime=1.38600138600139e-08
  adder : Sum  OutDataTypeStr=fixdt(1, 18, 8)  AccumDataTypeStr=fixdt(1, 18, 8)  SaturateOnIntegerOverflow=on  SampleTime=1.38600138600139e-08
  buffSig_bypass : Subsystem
  buffSig_bypass1 : Subsystem
  counter : Subsystem
  delayMatch_absorbed : Delay  DelayLength=0
  dtc : DataTypeConversion  OutDataTypeStr=fixdt(1, 18, 8)  ConvertRealWorld=Stored Integer (SI)  SampleTime=1.38600138600139e-08  RndMeth=Floor
  dtc1 : DataTypeConversion  OutDataTypeStr=fixdt(1, 18, 0)  ConvertRealWorld=Stored Integer (SI)  SampleTime=1.38600138600139e-08  RndMeth=Floor
  enb_counter_eq_0 : simulink/Logic and Bit Operations/Compare To Constant  relop===  const=double(0)  OutDataTypeStr=boolean
  enb_counter_eq_5 : simulink/Logic and Bit Operations/Compare To Constant  relop===  const=double(5)  OutDataTypeStr=boolean
  enb_counter_ge_32 : simulink/Logic and Bit Operations/Compare To Constant  relop=>=  const=double(32)  OutDataTypeStr=boolean
  enb_counter_le_4 : simulink/Logic and Bit Operations/Compare To Constant  relop=<=  const=double(4)  OutDataTypeStr=boolean
  enb_counter_le_5 : simulink/Logic and Bit Operations/Compare To Constant  relop=<=  const=double(5)  OutDataTypeStr=boolean
  gain : Gain  Gain="fi(0,0,1,4,\"hex\",\"1\")"  ParamDataTypeStr=fixdt(0, 1, 4)  OutDataTypeStr=fixdt(1, 18, 0)  SaturateOnIntegerOverflow=on  SampleTime=1.38600138600139e-08
  rd_0 : Delay  DelayLength=double(27)  InitialCondition=0  SampleTime=1.38600138600139e-08
  rd_1 : Delay  DelayLength=double(27)  InitialCondition=0  SampleTime=1.38600138600139e-08
  rd_2 : Delay  DelayLength=double(27)  InitialCondition=0  SampleTime=1.38600138600139e-08
  rd_3 : Delay  DelayLength=double(2)  InitialCondition=0  SampleTime=1.38600138600139e-08
  rd_4 : Delay  DelayLength=double(32)  InitialCondition=0  SampleTime=1.38600138600139e-08
  rd_5 : Delay  DelayLength=double(32)  InitialCondition=0  SampleTime=1.38600138600139e-08
  t : Mux  Inputs=2
  t1 : Mux  Inputs=2
  tappedDelay : Subsystem
  tappedDelay1 : Subsystem
  out0 : Outport  OutDataTypeStr=fixdt(1, 18, 8)  PortDimensions=[6]  SampleTime=1.38600138600139e-08
  out1 : Outport  Port=2  OutDataTypeStr=fixdt(1, 18, 8)  PortDimensions=[6]  SampleTime=1.38600138600139e-08
  wires:
  t/1 -> out0/1
  enb_counter_eq_0/1 -> Discrete-Time Integrator_u_sat_bypass1/2(in1), Discrete-Time Integrator_u_sat_bypass/2(in1)
  dtc/1 -> adder/2
  dtc1/1 -> gain/1
  Subtract/1 -> dtc1/1
  rd_4/1 -> adder/1
  Discrete-Time Integrator_u_sat_bypass1/1(out0) -> t/2
  HwModeRegister2/1 -> Multiply-Add/3
  HwModeRegister/1 -> Multiply-Add/1
  Subtract1/1 -> HwModeRegister/1
  rd_3/1 -> HwModeRegister1/1
  Gain1_out_dtc/1 -> Subtract1/1
  PipelineRegister2/1 -> Gain3_out_dtc/1
  PipelineRegister1/1 -> Gain1_out_dtc/1
  gain/1 -> dtc/1
  t1/1 -> out1/1
  delayMatch_absorbed/1 -> rd_3/1
  enb_counter_ge_32/1 -> tappedDelay/Enable
  OR/1 -> delayMatch_absorbed/1
  Gain1/1 -> PipelineRegister1/1
  buffSig_bypass/1(out0) -> t1/1
  Gain3_out_dtc/1 -> Subtract1/2, HwModeRegister2/1
  HwModeRegister6/1 -> Gain3/2
  HwModeRegister5/1 -> Gain3/1
  Discrete-Time Integrator_u_sat_bypass/1(out0) -> t/1
  rd_2/1 -> OR/1
  HwModeRegister4/1 -> Gain1/2
  adder/1 -> Discrete-Time Integrator_saturate/1
  HwModeRegister3/1 -> Gain1/1
  buffSig_bypass1/1(out0) -> t1/2
  tappedDelay1/1(out0) -> buffSig_bypass/1(in0)
  Equal/1 -> OR/2
  Serializer_Subnetwork2/1(out0) -> HwModeRegister5/1, Equal/2
  Constant/1 -> Equal/1
  Gain3_const/1 -> HwModeRegister6/1
  Gain1_const/1 -> HwModeRegister4/1
  Serializer_Subnetwork3/1(out0) -> HwModeRegister3/1
  Multiply-Add/1 -> PipelineRegister/1
  enb_counter_eq_5/1 -> buffSig_bypass1/2(in1), buffSig_bypass/2(in1)
  Serializer_Subnetwork/1(out0) -> buffSig_bypass1/1(in0), tappedDelay1/1(in0), rd_5/1, rd_4/1
  in2/1 -> Serializer_Subnetwork2/1(in0)
  Serializer_Subnetwork1/1(out0) -> rd_2/1
  rd_0/1 -> Serializer_Subnetwork3/2(in1)
  Discrete-Time Integrator_saturate/1 -> Discrete-Time Integrator_u_sat_bypass1/1(in0), tappedDelay/1(in0)
  in3/1 -> Serializer_Subnetwork3/1(in0)
  counter/1(out0) -> Serializer_Subnetwork/2(in1), Serializer_Subnetwork1/2(in1), rd_0/1, rd_1/1
  in1/1 -> Serializer_Subnetwork1/1(in0)
  HwModeRegister1/1 -> Multiply-Add/2
  enb_counter_le_4/1 -> tappedDelay1/Enable
  in0/1 -> Serializer_Subnetwork/1(in0)
  rd_1/1 -> Serializer_Subnetwork2/2(in1)
  rd_5/1 -> Subtract/2
  enb_counter_le_5/1 -> counter/Enable
  Gain3/1 -> PipelineRegister2/1
  PipelineRegister/1 -> Subtract/1
  tappedDelay/1(out0) -> Discrete-Time Integrator_u_sat_bypass/1(in0)
  enb_counter/1 -> enb_counter_le_4/1, enb_counter_le_5/1, enb_counter_eq_0/1, enb_counter_ge_32/1, enb_counter_eq_5/1

== system gm_HDL_pfc_gold_fi_og_vnl/simscape_system/simscape_system/HDL Subsystem/Sparse Matrix-Vector Product ==
  in0 : Inport  OutDataTypeStr=fixdt(1, 25, 13)  PortDimensions=[10]  SampleTime=1.38600138600139e-08
  selectSignal : Inport  Port=2  OutDataTypeStr=boolean  SampleTime=1.38600138600139e-08
  enb_counter : Inport  Port=3  OutDataTypeStr=fixdt(0, 6, 0)  SampleTime=1.38600138600139e-08
  SelectCols{1..6} (6 alike) : Selector  InputPortWidth=10  IndexOptions=Index vector (dialog)  Indices=double([2 3 4 5 6 7 8 9 10])  OutputSizes=double(1)
  SelectCols7 : Selector  InputPortWidth=10  IndexOptions=Index vector (dialog)  Indices=double([1 2 3 4 5 6 7 8 9])  OutputSizes=double(1)
  SelectRows1 : Selector  InputPortWidth=63  IndexOptions=Index vector (dialog)  Indices=double([2 9 16 23 30 37 44 51 58])  OutputSizes=double(1)
  SelectRows2 : Selector  InputPortWidth=63  IndexOptions=Index vector (dialog)  Indices=double([3 10 17 24 31 38 45 52 59])  OutputSizes=double(1)
  SelectRows3 : Selector  InputPortWidth=63  IndexOptions=Index vector (dialog)  Indices=double([4 11 18 25 32 39 46 53 60])  OutputSizes=double(1)
  SelectRows4 : Selector  InputPortWidth=63  IndexOptions=Index vector (dialog)  Indices=double([5 12 19 26 33 40 47 54 61])  OutputSizes=double(1)
  SelectRows5 : Selector  InputPortWidth=63  IndexOptions=Index vector (dialog)  Indices=double([6 13 20 27 34 41 48 55 62])  OutputSizes=double(1)
  SelectRows6 : Selector  InputPortWidth=63  IndexOptions=Index vector (dialog)  Indices=double([7 14 21 28 35 42 49 56 63])  OutputSizes=double(1)
  SelectRows7 : Selector  InputPortWidth=63  IndexOptions=Index vector (dialog)  Indices=double([1 8 15 22 29 36 43 50 57])  OutputSizes=double(1)
  concatenate : Concatenate  NumInputs=7
  configuration1_wire : hdlmdlgenlib/Buffer
  const : Constant  Value=[-0.0010908753611147403717041015625;0.0008385316468775272369384765625;-0.0004192660562694072723388671875;-0.0004192660562694072723388671875;-0.00041927397251129150390625;-0.00041927397251129150390625;0.0008385479450225830078125;0.0005454379133880138397216796875;-0.0008385316468775272369384765625;0.0004192660562694072723388671875;0.0004192660562694072723388671875;0.00041927397251129150390625;0.00041927397251129150390625;-0.0008385479450225830078125;0.0005454379133880138397216796875;0.0004192660562694072723388671875;-0.0008385316468775272369384765625;0.0004192660562694072723388671875;-0.0008385479450225830078125;0.00041927397251129150390625;0.00041927397251129150390625;0.0005454379133880138397216796875;0.0004192660562694072723388671875;0.0004192660562694072723388671875;-0.0008385316468775272369384765625;0.00041927397251129150390625;-0.0008385479450225830078125;0.00041927397251129150390625;0.0005454379133880138397216796875;-0.0004192660562694072723388671875;0.0008385316468775272369384765625;-0.0004192660562694072723388671875;0.0008385479450225830078125;-0.00041927397251129150390625;-0.00041927397251129150390625;0.0005454379133880138397216796875;-0.0004192660562694072723388671875;-0.0004192660562694072723388671875;0.0008385316468775272369384765625;-0.00041927397251129150390625;0.0008385479450225830078125;-0.00041927397251129150390625;0.0005454379133880138397216796875;3.35411168634891510009765625e-05;-1.67707912623882293701171875e-05;-1.67707912623882293701171875e-05;-1.67707912623882293701171875e-05;-1.67707912623882293701171875e-05;3.35420481860637664794921875e-05;0;-1.67707912623882293701171875e-05;3.35411168634891510009765625e-05;-1.67707912623882293701171875e-05;3.35420481860637664794921875e-05;-1.67707912623882293701171875e-05;-1.67707912623882293701171875e-05;0;-1.67707912623882293701171875e-05;-1.67707912623882293701171875e-05;3.35411168634891510009765625e-05;-1.67707912623882293701171875e-05;3.35420481860637664794921875e-05;-1.67707912623882293701171875e-05]  OutDataTypeStr=fixdt(1, 25, 31)  SampleTime=1.38600138600139e-08
  dtc{,1..6} (7 alike) : DataTypeConversion  OutDataTypeStr=fixdt(1, 25, 13)  RndMeth=Nearest  SampleTime=1.38600138600139e-08  SaturateOnIntegerOverflow=off
  hNNewMatrixB_shared : Subsystem
  rd_{0..6} (7 alike) : Delay  DelayLength=double(1)  InitialCondition=0  SampleTime=1.38600138600139e-08
  terminator : Terminator
  matrixBOutSignal : Outport  OutDataTypeStr=fixdt(1, 25, 13)  PortDimensions=[7]  SampleTime=1.38600138600139e-08
  wires:
  concatenate/1 -> matrixBOutSignal/1
  rd_6/1 -> concatenate/7
  rd_5/1 -> concatenate/6
  rd_3/1 -> concatenate/4
  rd_4/1 -> concatenate/5
  rd_2/1 -> concatenate/3
  rd_1/1 -> concatenate/2
  dtc/1 -> concatenate/1
  dtc6/1 -> rd_6/1
  dtc5/1 -> rd_5/1
  dtc4/1 -> rd_4/1
  dtc3/1 -> rd_3/1
  dtc1/1 -> rd_1/1
  dtc2/1 -> rd_2/1
  rd_0/1 -> dtc/1
  hNNewMatrixB_shared/7(out6) -> rd_0/1
  hNNewMatrixB_shared/6(out5) -> dtc1/1
  hNNewMatrixB_shared/5(out4) -> dtc2/1
  hNNewMatrixB_shared/4(out3) -> dtc3/1
  hNNewMatrixB_shared/3(out2) -> dtc4/1
  hNNewMatrixB_shared/2(out1) -> dtc5/1
  SelectRows1/1 -> hNNewMatrixB_shared/13(in12)
  SelectCols2/1 -> hNNewMatrixB_shared/12(in11)
  SelectCols1/1 -> hNNewMatrixB_shared/14(in13)
  SelectRows2/1 -> hNNewMatrixB_shared/11(in10)
  SelectCols3/1 -> hNNewMatrixB_shared/10(in9)
  SelectRows3/1 -> hNNewMatrixB_shared/9(in8)
  SelectCols4/1 -> hNNewMatrixB_shared/8(in7)
  SelectRows5/1 -> hNNewMatrixB_shared/5(in4)
  SelectRows4/1 -> hNNewMatrixB_shared/7(in6)
  SelectRows6/1 -> hNNewMatrixB_shared/3(in2)
  SelectCols7/1 -> hNNewMatrixB_shared/2(in1)
  SelectRows7/1 -> hNNewMatrixB_shared/1(in0)
  hNNewMatrixB_shared/1(out0) -> dtc6/1
  SelectCols6/1 -> hNNewMatrixB_shared/4(in3)
  in0/1 -> SelectCols7/1, SelectCols1/1, SelectCols6/1, SelectCols3/1, SelectCols2/1, SelectCols4/1, SelectCols5/1
  selectSignal/1 -> terminator/1
  SelectCols5/1 -> hNNewMatrixB_shared/6(in5)
  enb_counter/1 -> hNNewMatrixB_shared/15(enb_counter)
  const/1 -> configuration1_wire/1
  configuration1_wire/1 -> SelectRows1/1, SelectRows5/1, SelectRows4/1, SelectRows2/1, SelectRows3/1, SelectRows6/1, SelectRows7/1

== system gm_HDL_pfc_gold_fi_og_vnl/simscape_system/simscape_system/HDL Subsystem/Sparse Matrix-Vector Product1 ==
  delayOutSignal : Inport  OutDataTypeStr=fixdt(1, 25, 13)  PortDimensions=[7]  SampleTime=1.38600138600139e-08
  selectSignal : Inport  Port=2  OutDataTypeStr=boolean  SampleTime=1.38600138600139e-08
  enb_counter : Inport  Port=3  OutDataTypeStr=fixdt(0, 6, 0)  SampleTime=1.38600138600139e-08
  SelectCols{1..6} (6 alike) : Selector  InputPortWidth=7  IndexOptions=Index vector (dialog)  Indices=double([1 2 3 4 5 6])  OutputSizes=double(1)
  SelectCols7 : Selector  InputPortWidth=7  IndexOptions=Index vector (dialog)  Indices=double([1 2 3 4 5 7])  OutputSizes=double(1)
  SelectRows1 : Selector  InputPortWidth=42  IndexOptions=Index vector (dialog)  Indices=double([1 8 15 22 29 36])  OutputSizes=double(1)
  SelectRows2 : Selector  InputPortWidth=42  IndexOptions=Index vector (dialog)  Indices=double([2 9 16 23 30 37])  OutputSizes=double(1)
  SelectRows3 : Selector  InputPortWidth=42  IndexOptions=Index vector (dialog)  Indices=double([3 10 17 24 31 38])  OutputSizes=double(1)
  SelectRows4 : Selector  InputPortWidth=42  IndexOptions=Index vector (dialog)  Indices=double([4 11 18 25 32 39])  OutputSizes=double(1)
  SelectRows5 : Selector  InputPortWidth=42  IndexOptions=Index vector (dialog)  Indices=double([5 12 19 26 33 40])  OutputSizes=double(1)
  SelectRows6 : Selector  InputPortWidth=42  IndexOptions=Index vector (dialog)  Indices=double([6 13 20 27 34 41])  OutputSizes=double(1)
  SelectRows7 : Selector  InputPortWidth=42  IndexOptions=Index vector (dialog)  Indices=double([7 14 21 28 35 42])  OutputSizes=double(1)
  concatenate : Concatenate  NumInputs=7
  configuration1_wire : hdlmdlgenlib/Buffer
  const : Constant  Value=[0.6540615558624267578125;-0.327021062374114990234375;-0.327021062374114990234375;-0.32702732086181640625;-0.32702732086181640625;0.654054582118988037109375;0;-0.327021062374114990234375;0.6540615558624267578125;-0.327021062374114990234375;0.654054582118988037109375;-0.32702732086181640625;-0.32702732086181640625;0;-0.327021062374114990234375;-0.327021062374114990234375;0.6540615558624267578125;-0.32702732086181640625;0.654054582118988037109375;-0.32702732086181640625;0;-0.005886495113372802734375;0.01177299022674560546875;-0.005886495113372802734375;0.011773586273193359375;-0.005886614322662353515625;-0.005886614322662353515625;0;-0.005886495113372802734375;-0.005886495113372802734375;0.01177299022674560546875;-0.005886614322662353515625;0.011773586273193359375;-0.005886614322662353515625;0;0.01177299022674560546875;-0.005886495113372802734375;-0.005886495113372802734375;-0.005886614322662353515625;-0.005886614322662353515625;0.011773586273193359375;0.999967277050018310546875]  OutDataTypeStr=fixdt(1, 25, 24)  SampleTime=1.38600138600139e-08
  dtc{,1..6} (7 alike) : DataTypeConversion  OutDataTypeStr=fixdt(1, 25, 13)  RndMeth=Nearest  SampleTime=1.38600138600139e-08  SaturateOnIntegerOverflow=off
  hNNewMatrixA_shared : Subsystem
  terminator : Terminator
  matrixAOutSignal : Outport  OutDataTypeStr=fixdt(1, 25, 13)  PortDimensions=[7]  SampleTime=1.38600138600139e-08
  wires:
  concatenate/1 -> matrixAOutSignal/1
  dtc6/1 -> concatenate/7
  dtc4/1 -> concatenate/5
  hNNewMatrixA_shared/7(out6) -> dtc/1
  dtc2/1 -> concatenate/3
  hNNewMatrixA_shared/6(out5) -> dtc1/1
  hNNewMatrixA_shared/5(out4) -> dtc2/1
  hNNewMatrixA_shared/4(out3) -> dtc3/1
  hNNewMatrixA_shared/3(out2) -> dtc4/1
  hNNewMatrixA_shared/1(out0) -> dtc6/1
  SelectRows1/1 -> hNNewMatrixA_shared/13(in12)
  dtc5/1 -> concatenate/6
  SelectCols2/1 -> hNNewMatrixA_shared/12(in11)
  SelectCols3/1 -> hNNewMatrixA_shared/10(in9)
  SelectCols1/1 -> hNNewMatrixA_shared/14(in13)
  hNNewMatrixA_shared/2(out1) -> dtc5/1
  SelectRows3/1 -> hNNewMatrixA_shared/9(in8)
  dtc3/1 -> concatenate/4
  SelectCols4/1 -> hNNewMatrixA_shared/8(in7)
  SelectCols5/1 -> hNNewMatrixA_shared/6(in5)
  dtc/1 -> concatenate/1
  SelectRows5/1 -> hNNewMatrixA_shared/5(in4)
  SelectRows6/1 -> hNNewMatrixA_shared/3(in2)
  SelectRows7/1 -> hNNewMatrixA_shared/1(in0)
  enb_counter/1 -> hNNewMatrixA_shared/15(enb_counter)
  delayOutSignal/1 -> SelectCols1/1, SelectCols2/1, SelectCols3/1, SelectCols7/1, SelectCols4/1, SelectCols6/1, SelectCols5/1
  SelectRows2/1 -> hNNewMatrixA_shared/11(in10)
  SelectCols6/1 -> hNNewMatrixA_shared/4(in3)
  dtc1/1 -> concatenate/2
  SelectCols7/1 -> hNNewMatrixA_shared/2(in1)
  configuration1_wire/1 -> SelectRows1/1, SelectRows7/1, SelectRows3/1, SelectRows2/1, SelectRows4/1, SelectRows5/1, SelectRows6/1
  const/1 -> configuration1_wire/1
  selectSignal/1 -> terminator/1
  SelectRows4/1 -> hNNewMatrixA_shared/7(in6)
